simulink model "quarter_car"  (R2024b)
settings: Solver=VariableStepAuto  StartTime=0.0  StopTime=10  MaxStep=1e-3  RelTol=1e-3
PreLoadFcn:
  | proj = fileparts(fileparts(get_param(bdroot,'FileName')));
  | addpath(fullfile(proj, 'matlab'));
  | addpath(fullfile(proj, 'adams'));
  | init
undefined symbols (not defined in the file): ADAMS_communication_interval, ADAMS_communications_per_output_step, ADAMS_cwd, ADAMS_exec, ADAMS_host, ADAMS_init, ADAMS_inputs, ADAMS_outputs, ADAMS_pinput_id, ADAMS_poutput_id, ADAMS_prefix, ADAMS_static, ADAMS_sysdir, ADAMS_time_offset, cs_p, cs_s, use_random, use_skyhook
settings Model: Creator=Remote  LastModifiedBy=Remote
settings DataIOCC: OutputOption=SpecifiedOutputTimes  OutputTimes=0:0.001:10

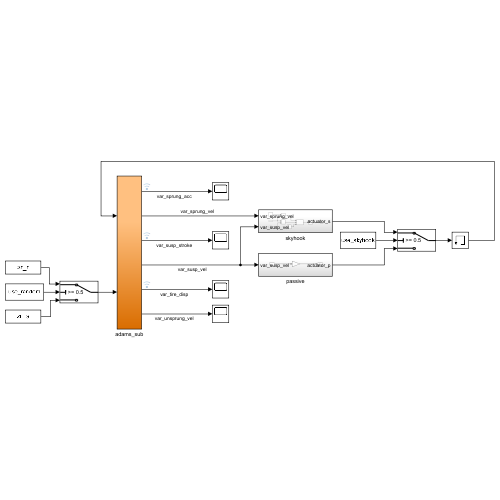
[thumbnail: Simulink's stored preview of the top-level diagram]
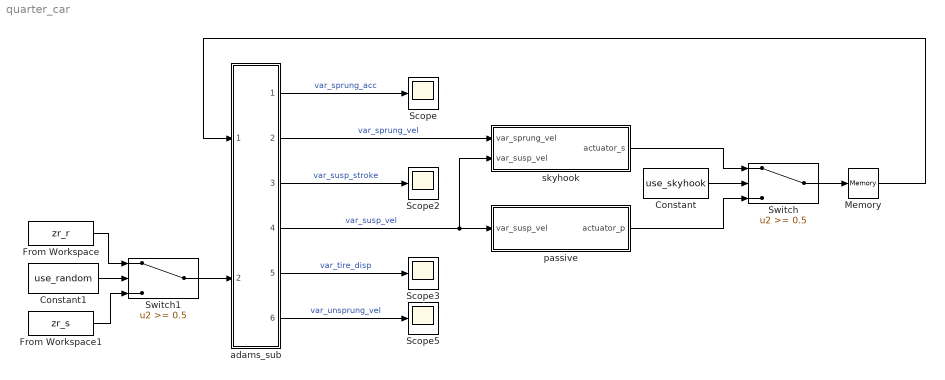
== system quarter_car ==
  Constant : Constant  Value=use_skyhook
  Constant1 : Constant  Value=use_random
  From Workspace : FromWorkspace  VariableName=zr_r
  From Workspace1 : FromWorkspace  VariableName=zr_s
  Memory : Memory
  Scope{,2..3,5} (4 alike) : Scope
  Switch : Switch  Threshold=0.5  SaturateOnIntegerOverflow=off  InputSameDT=off
  Switch1 : Switch  Threshold=0.5  SaturateOnIntegerOverflow=off  InputSameDT=off
  adams_sub : Subsystem
  passive : Subsystem
  skyhook : Subsystem
  wires:
  adams_sub/6(var_unsprung_vel) -> Scope5/1  "var_unsprung_vel"
  adams_sub/3("var_susp_stroke ") -> Scope2/1  "var_susp_stroke"
  adams_sub/5("var_tire_disp   ") -> Scope3/1  "var_tire_disp"
  adams_sub/4("var_susp_vel    ") -> skyhook/2(var_susp_vel), passive/1(var_susp_vel)  "var_susp_vel"
  adams_sub/2("var_sprung_vel  ") -> skyhook/1(var_sprung_vel)  "var_sprung_vel"
  adams_sub/1("var_sprung_acc  ") -> Scope/1  "var_sprung_acc"
  skyhook/1(actuator_s) -> Switch/1
  Constant/1 -> Switch/2
  passive/1(actuator_p) -> Switch/3
  Switch/1 -> Memory/1
  Memory/1 -> adams_sub/1("var_actuator ")
  Constant1/1 -> Switch1/2
  From Workspace1/1 -> Switch1/3
  From Workspace/1 -> Switch1/1
  Switch1/1 -> adams_sub/2(var_road_disp)

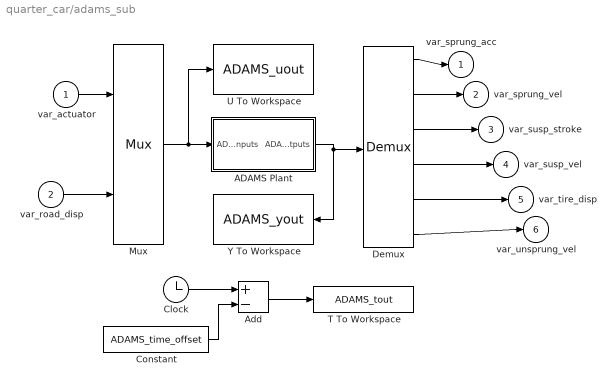
== system quarter_car/adams_sub ==
  "var_actuator " : Inport
  var_road_disp : Inport  Port=2
  ADAMS Plant : Subsystem  LoadFcn=|  InitFcn=clear mex  mask(Adams Plant){exevie=ADAMS_sysdir, nam_in=ADAMS_inputs, namout=ADAMS_outputs, nampre=ADAMS_prefix, outfil=ADAMS_prefix, exesol=ADAMS_exec, stat=ADAMS_static, inicmd=[ADAMS_init], exetyp=C++, comtyp=PIPE(DDE), workdir=ADAMS_cwd, ada_host=ADAMS_host, modani=batch, modsim=discrete, dft=no, simulink_lead_cosim=yes, pin_interp_order=0, pout_extrap_order=0, pin_extrap_order=0, pout_interp_order=0, dt_out=ADAMS_communication_interval, o_rate=ADAMS_communications_per_output_step, time_offset=ADAMS_time_offset, pinput_id=ADAMS_pinput_id, poutput_id=ADAMS_poutput_id, more=on}
      | %check based on dialog box setting for when setting by popup menu                                             
      | if exist('ADAMS_solver_type')                                                                                 
      |   if strcmp(ADAMS_solver_type,'C++')                                                                          
      |     set_param(gcb,'exetyp','C++');                                                                            
      |   else                                                                                                        
      |     set_param(gcb,'exetyp','Fortran');                                                                        
      |   end                                                                                                         
      | else                                                                                                          
      |   set_param(gcb,'exetyp','C++');                                                                              
      | end                                                                                                           
      | %set the mode if using acar_solver                                                                            
      | %REQUIRED HERE BECAUSE BELOW CAUSES MDLTERMINATE TO BE CALLED 2 TIMES IN MIDDLE OF SIMULATION WHEN SET IN MASK
      |                                                                                                               
      | %enable the direct feedthrough, sim mode, anim mode parameters by default                                     
      |                                                                                                               
      | if exist('set_some_params_states')                                                                            
      |                                                                                                               
      |   set_some_params_states({'dft','modsim','modani'},{'on','on','on'},'MaskEnables',gcb)                        
      |   %turn on direct feedthrough option                                                                          
      |   set_some_params_states({'dft'},{'on'},'MaskVisibilities',gcb)                                               
      |                                                                                                               
      |  end                                                                                                          
      |                                                                                                               
      |                                                                                                               
      | if exist('ADAMS_exec')                                                                                        
      |   if and(strcmp(get_param(gcb,'exesol'),'ADAMS_exec'),strcmp(ADAMS_exec,'acar_solver'))                       
      |     %set the sim mode to discrete -- only supported mode                                                      
      |     set_param(gcb,'modsim','discrete')                                                                        
      |      %turn off direct feedthrough option                                                                      
      |      set_some_params_states({'dft'},{'off'},'MaskVisibilities',gcb)                                           
      |     %set the animation mode to batch -- only supported mode                                                   
      |     set_param(gcb,'modani','batch')                                                                           
      |     %disable the direct feedthrough, sim mode, anim mode parameters                                           
      |     set_some_params_states({'modsim','modani'},{'off','off'},'MaskEnables',gcb)                               
      |   end
      |   if and(strcmp(get_param(gcb,'exesol'),'ADAMS_exec'),strcmp(ADAMS_exec,'apre_solver'))                       
      |     %set the sim mode to discrete -- only supported mode                                                      
      |     set_param(gcb,'modsim','discrete')                                                                        
      |      %turn off direct feedthrough option                                                                      
      |      set_some_params_states({'dft'},{'off'},'MaskVisibilities',gcb)                                           
      |     %set the animation mode to batch -- only supported mode                                                   
      |     set_param(gcb,'modani','batch')                                                                           
      |     %disable the direct feedthrough, sim mode, anim mode parameters                                           
      |     set_some_params_states({'modsim','modani'},{'off','off'},'MaskEnables',gcb)                               
      |   end                                                                                                  
      | end
      mask prompts: exevie "Adams install directory"; nam_in "Adams View input names"; namout "Adams View output names"; nampre "Adams model file prefix"; outfil "Output files prefix (opt.: if blank - no output)"; exesol "User executable (opt.: if blank - use standard)"; stat "Initial static simulation flag"; inicmd "Initialization commands"; exetyp "Adams Solver type"; comtyp "Interprocess option"; workdir "Adams working directory"; ada_host "Adams host"; modani "Animation mode"; modsim "Simulation mode"; dft "Direct feedthrough"; simulink_lead_cosim "Discrete Computational Order - Simulink Leads Adams"; pin_interp_order "Plant input interpolation order"; pout_extrap_order "Plant output extrapolation order"; pin_extrap_order "Plant input extrapolation order"; pout_interp_order "Plant output interpolation order"; dt_out "Communication interval"; o_rate "Number of communications per output step"; time_offset "Offset between Simulink and Adams simulation time"; pinput_id "Plant Input ID"; poutput_id "Plant Output ID"; more "More parameters"
      mask help: Simulate any Adams plant model either in Adams Solver form (.adm file) or in Adams View form (.cmd file)
      settings: OpenFcn=|
      | open_system(gcb,'mask')
      | if not(exist('set_some_params_states'))
      | 
      | warning('The script "set_some_params_states.m" cannot be found in the MATLAB PATH.  Cannot update the ADAMS Plant S-Function parameters.')
      | 
      | warning('Recommended action(optional):  run the Adams Controls .m file first to help choose the correct settings in the Adams S-Function block.')
      | 
      | end
      mask Help:
      | <html>
      | This S-Function represents the non-linear Adams Plant with the inputs sent to the Adams model as input #1 and Time as input #2<br>
      |  and the outputs generated by the Adams model.  See the Adams Controls documentation for more <br>
      | information.  This plant uses the following variables:<br>
      | <br>
      | <b>ADAMS_sysdir:</b> Adams installation directory<br>
      | <b>ADAMS_inputs:</b> Input variables View names vector<br>
      | <b>ADAMS_outputs :</b> Outputs variables View names vector<br>
      | <b>ADAMS_prefix:</b> ADAMS model files prefix (.adm, .cmd); also doubles as output files prefix<br>
      | <b>ADAMS_exec:</b>  Adams Solver user library or keyword (e.g., acar_solver)<br>
      | <b>ADAMS_static:</b> yes|no - initial static before Co-simulation(discrete)/Function Evaluation(continuous)<br>
      | <b>ADAMS_init:</b> Initialization commands (i.e., Adams View or Solver commands, depending on setting for Animation mode)<br>
      | <b>ADAMS_cwd:</b> Current working directory (for TCP/IP)<br>
      | <b>ADAMS_host:</b> Name of Adams server host (for TCP/IP)<br>
      | <b>ADAMS_mode:</b> Linear or non-linear (i.e., co-sim, function eval)<br>
      | <b>ADAMS_solver_type:</b> Fortran or C++ (used to set popup menu when first loaded)<br>
      | <b>ADAMS_communication_interval:</b> Time step at which Co-simulation exchange information (e.g.,0.005); also controls <br>output for continuous mode (Function Evaluation)<br>
      | <b>ADAMS_communications_per_output_step: </b>Sets Adams output rate (.res, .req, .gra) integer value (default: 1)<br>
      | <b>ADAMS_time_offset: </b>Removes this time offset from simulation time used by Adams. Adams will be sent a time value being Simulink simulation time - this value. (default: 0). Eg. if ADAMS_time_offset=2: if Simulink time=2 then Adams time = 0. Make sure that the Adams block is disabled when the Adams time is <0. If not an error will be raised. <br>
      | 
      | 
      | <br>
      | The following settings can be chosen:<br>
      | <br>
      | <b>Adams Solver type:</b>  Fortran or C++ (will also set ADAMS_solver_type)<br>
      | <b>Interprocess option:</b> Pipe(DDE), TCP/IP or DIRECT; TCP/IP can allow different machines run Adams and MATLAB<br>
      | <b>Animation mode:</b> batch (Solver, uses .adm) or interactive (View, uses .cmd)<br>
      | <b>Simulation mode:</b> discrete (Co-simulation) or continuous (Function Evaluation)<br>
      | <b>Discrete Computational Order - Simulink Lead Adams:</b> for discrete mode, chooses if Simulink leads the integration (yes) or lags (no);<br> if set to "no", can remove algebraic loop<br>
      | <b>Plant input interpolation order:</b> 0 = zero-order hold; 1 = linear (discrete mode only, where Simulink leads)<br>
      | <b>Plant output extrapolation order:</b> 0 = zero-order hold;1 = linear(discrete mode only, where Simulink leads)<br>
      | <b>Plant input extrapolation order:</b> 0 = zero-order hold; 1 = linear (discrete mode only, where Adams leads)<br>
      | <b>Plant output interpolation order:</b> 0 = zero-order hold;1 = linear(discrete mode only, where Adams leads)<br>
      | <b>Direct feedthrough:</b> yes|no - yes = Input directly effect output(continuous mode-only)<br>
      | 
      | </html>
      mask Callback exesol:
      | if exist('set_some_params_states')
      | %enable the direct feedthrough, sim mode, anim mode parameters
      | set_some_params_states({'dft','modsim','modani'},{'on','on','on'},'MaskEnables',gcb)
      | %turn on direct feedthrough option
      | set_some_params_states({'dft'},{'on'},'MaskVisibilities',gcb)
      | end
      | 
      | if exist('ADAMS_exec')
      |   if and(strcmp(get_param(gcb,'exesol'),'ADAMS_exec'),strcmp(ADAMS_exec,'acar_solver'))
      |     %set the sim mode to discrete -- only supported mode
      |     %REMOVED:  BELOW CAUSES MDLTERMINATE TO BE CALLED 2 TIMES IN MIDDLE OF SIMULATION
      |     %Now in LoadFcn callback
      |     %set_param(gcb,'modsim','discrete')
      |      %turn off direct feedthrough option
      |     set_some_params_states({'dft'},{'off'},'MaskVisibilities',gcb)
      |     %set the animation mode to batch -- only supported mode
      |     %REMOVED:  BELOW CAUSES MDLTERMINATE TO BE CALLED 2 TIMES IN MIDDLE OF SIMULATION
      |     %Now in LoadFcn callback
      |     %set_param(gcb,'modani','batch')
      |     %disable the direct feedthrough, sim mode, anim mode parameters
      |     set_some_params_states({'modsim','modani'},{'off','off'},'MaskEnables',gcb)
      |   end
      | end
      mask TypeOptions exetyp: Fortran | C++
      mask Callback exetyp:
      | if strcmp(get_param(gcb,'exetyp'),'C++')
      |     ADAMS_solver_type='C++';
      | else
      |     ADAMS_solver_type='Fortran';
      | end
      mask TypeOptions comtyp: PIPE(DDE) | TCP/IP | DIRECT
      mask Callback comtyp:
      | if exist('set_some_params_states')
      | if strcmp(get_param(gcb,'comtyp'),'PIPE(DDE)') || strcmp(get_param(gcb,'comtyp'),'DIRECT')
      |     %turn off cwd, host options
      |     set_some_params_states({'ada_host','workdir'},{'off','off'},'MaskVisibilities',gcb)
      | else%if strcmp(get_param(gcb,'modsim'),'TCP/IP')
      |     %turn on cwd, host options
      |     set_some_params_states({'ada_host','workdir'},{'on','on'},'MaskVisibilities',gcb)
      | end
      | end
      mask TypeOptions modani: batch | interactive
      mask TypeOptions modsim: discrete | continuous
      mask Callback modsim:
      | if exist('set_some_params_states')
      | if strcmp(get_param(gcb,'modsim'),'discrete')
      |      %turn off direct feedthrough option
      |     set_some_params_states({'dft'},{'off'},'MaskVisibilities',gcb)
      |     %turn on discrete co-sim type if want to see more
      |     if strcmp(get_param(gcb,'more'),'on')
      |         set_some_params_states({'simulink_lead_cosim'},{'on'},'MaskVisibilities',gcb)
      |     end
      |     if strcmp(get_param(gcb,'simulink_lead_cosim'),'yes')
      |         %turn on interpolation/extrapolation options
      |         set_some_params_states({'pin_interp_order','pout_extrap_order',},{'on','on'},'MaskVisibilities',gcb)
      |     else
      |         set_some_params_states({'pin_extrap_order','pout_interp_order'},{'on','on'},'MaskVisibilities',gcb)
      |     end
      | else%if strcmp(get_param(gcb,'modsim'),'continuous')
      |      %turn off direct feedthrough option
      |     set_some_params_states({'dft'},{'on'},'MaskVisibilities',gcb)
      |     %turn off interpolation/extrapolation options
      |     set_some_params_states({'pin_interp_order','pout_extrap_order','pin_extrap_order','pout_interp_order','simulink_lead_cosim'},{'off','off','off','off','off'},'MaskVisibilities',gcb)
      | end
      | end
      mask TypeOptions dft: no | yes
      mask TypeOptions simulink_lead_cosim: yes | no
      mask Callback simulink_lead_cosim:
      | if exist('set_some_params_states')
      | if (strcmp(get_param(gcb,'simulink_lead_cosim'),'yes') && strcmp(get_param(gcb,'modsim'),'discrete'))
      |      %turn off unused interpolate/extrapolate options
      |     set_some_params_states({'pin_extrap_order','pout_interp_order'},{'off','off'},'MaskVisibilities',gcb)
      |     %turn on used interpolate/extrapolate options
      |     set_some_params_states({'pin_interp_order','pout_extrap_order'},{'on','on'},'MaskVisibilities',gcb)
      | elseif (strcmp(get_param(gcb,'simulink_lead_cosim'),'no') && strcmp(get_param(gcb,'modsim'),'discrete'))
      |     %turn on used interpolate/extrapolate options
      |     set_some_params_states({'pin_extrap_order','pout_interp_order'},{'on','on'},'MaskVisibilities',gcb)
      |      %turn off unused interpolate/extrapolate options
      |     set_some_params_states({'pin_interp_order','pout_extrap_order'},{'off','off'},'MaskVisibilities',gcb)
      | end
      | end
      mask TypeOptions pin_interp_order: 0 | 1
      mask TypeOptions pout_extrap_order: 0 | 1
      mask TypeOptions pin_extrap_order: 0 | 1
      mask TypeOptions pout_interp_order: 0 | 1
      mask Callback more:
      | if exist('set_some_params_states')
      | if (strcmp(get_param(gcb,'more'),'on'))
      |      %turn on infrequently used options
      |     set_some_params_states({'exevie','nam_in','namout','exesol','stat','inicmd','time_offset'},{'on','on','on','on','on','on','on'},'MaskVisibilities',gcb)
      |     if strcmp(get_param(gcb,'modsim'),'discrete')
      |         set_some_params_states({'simulink_lead_cosim'},{'on'},'MaskVisibilities',gcb)
      |     end
      | elseif (strcmp(get_param(gcb,'more'),'off'))
      |     %turn off infrequently used options
      |     set_some_params_states({'exevie','nam_in','namout','exesol','stat','inicmd','time_offset'},{'off','off','off','off','off','off','off'},'MaskVisibilities',gcb)
      |     if strcmp(get_param(gcb,'modsim'),'discrete')
      |         set_some_params_states({'simulink_lead_cosim'},{'off'},'MaskVisibilities',gcb)
      |     end
      | end
      | end
      mask Display: disp( 'MSC Software' )
  Add : Sum  Inputs=+-
  Clock : Clock
  Constant : Constant  Value=ADAMS_time_offset
  Demux : Demux  Outputs=6
      settings: DisplayOption=none
  Mux : Mux  Inputs=2
  T To Workspace : ToWorkspace  VariableName=ADAMS_tout
      settings: MaxDataPoints=100000
  U To Workspace : ToWorkspace  VariableName=ADAMS_uout
      settings: MaxDataPoints=100000
  Y To Workspace : ToWorkspace  VariableName=ADAMS_yout
      settings: MaxDataPoints=100000
  "var_sprung_acc  " : Outport
  "var_sprung_vel  " : Outport  Port=2
  "var_susp_stroke " : Outport  Port=3
  "var_susp_vel    " : Outport  Port=4
  "var_tire_disp   " : Outport  Port=5
  var_unsprung_vel : Outport  Port=6
  wires:
  Mux/1 -> ADAMS Plant/1(ADAMS inputs), U To Workspace/1
  ADAMS Plant/1(ADAMS outputs) -> Demux/1, Y To Workspace/1
  Clock/1 -> Add/1
  Constant/1 -> Add/2
  Add/1 -> T To Workspace/1
  Demux/1 -> "var_sprung_acc  "/1
  Demux/2 -> "var_sprung_vel  "/1
  Demux/3 -> "var_susp_stroke "/1
  Demux/4 -> "var_susp_vel    "/1
  Demux/5 -> "var_tire_disp   "/1
  Demux/6 -> var_unsprung_vel/1
  "var_actuator "/1 -> Mux/1
  var_road_disp/1 -> Mux/2

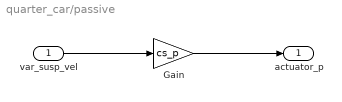
== system quarter_car/passive ==
  var_susp_vel : Inport
  Gain : Gain  Gain=cs_p
  actuator_p : Outport
  wires:
  var_susp_vel/1 -> Gain/1
  Gain/1 -> actuator_p/1

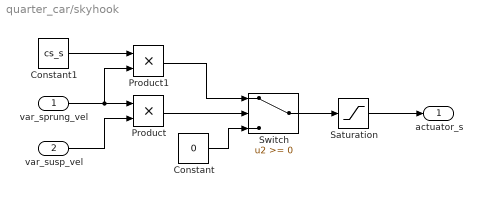
== system quarter_car/skyhook ==
  var_sprung_vel : Inport
  var_susp_vel : Inport  Port=2
  Constant : Constant  Value=0
  Constant1 : Constant  Value=cs_s
  Product : Product
  Product1 : Product
  Saturation : Saturate  UpperLimit=3000  LowerLimit=-3000
  Switch : Switch  SaturateOnIntegerOverflow=off  InputSameDT=off
  actuator_s : Outport
  wires:
  var_sprung_vel/1 -> Product1/2, Product/1
  var_susp_vel/1 -> Product/2
  Product/1 -> Switch/2
  Constant/1 -> Switch/3
  Constant1/1 -> Product1/1
  Product1/1 -> Switch/1
  Switch/1 -> Saturation/1
  Saturation/1 -> actuator_s/1

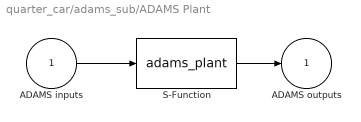
== system quarter_car/adams_sub/ADAMS Plant ==
  ADAMS inputs : Inport
  S-Function : S-Function  StopFcn=clear mex  FunctionName=adams_plant  Parameters=exevie,exesol,stat,outfil,nampre,o_rate,nam_in,namout,dft,modsim,modani,dt_out,inicmd,exetyp,comtyp,ada_host, workdir,pin_interp_order,pout_extrap_order,pin_extrap_order,pout_interp_order,simulink_lead_cosim,time_offset,pinput_id,poutput_id  SFunctionDeploymentMode=off  EnableBusSupport=off
  ADAMS outputs : Outport  InitialOutput=0  VectorParamsAs1DForOutWhenUnconnected=off
  wires:
  ADAMS inputs/1 -> S-Function/1
  S-Function/1 -> ADAMS outputs/1
